simulink model "determinarTiemposYDistanciasEnAceleracion"  (R2017a)
settings: Solver=FixedStepAuto  StartTime=0.0  StopTime=15  FixedStep=0.001  RelTol=1e-3
values from neighbouring files (symbols this model uses):
  vmaxh = 3    [operacionAutomatica.m]
  vmaxt = 4    [operacionAutomatica.m]
undefined symbols (not defined in the file or in its folder): vmaxhfull
settings Model: Creator=yellow submarine  LastModifiedBy=yellow submarine

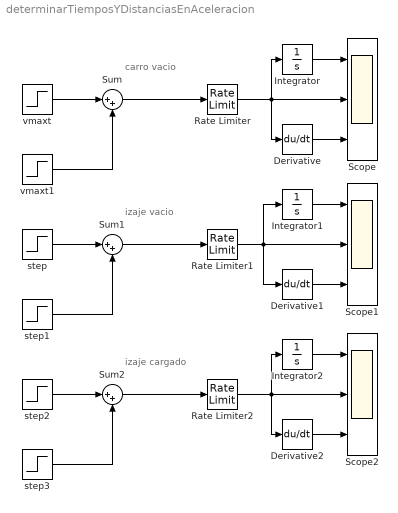
== system determinarTiemposYDistanciasEnAceleracion ==
  note: carro vacio
  note: izaje vacio
  note: izaje cargado
  Derivative : Derivative
  Derivative1 : Derivative
  Derivative2 : Derivative
  Integrator : Integrator
  Integrator1 : Integrator
  Integrator2 : Integrator
  Rate Limiter : RateLimiter
  Rate Limiter1 : RateLimiter
  Rate Limiter2 : RateLimiter
  Scope : Scope  NumInputPorts=3
  Scope1 : Scope  NumInputPorts=3
  Scope2 : Scope  NumInputPorts=3
  Sum : Sum  Inputs=|++
  Sum1 : Sum  Inputs=|++
  Sum2 : Sum  Inputs=|++
  step : Step  Time=.1  After=vmaxh  SampleTime=0
  step1 : Step  Time=3.1  After=-vmaxh  SampleTime=0
  step2 : Step  Time=.1  After=vmaxhfull  SampleTime=0
  step3 : Step  Time=1.6  After=-vmaxhfull  SampleTime=0
  vmaxt : Step  Time=.1  After=vmaxt  SampleTime=0
  vmaxt1 : Step  Time=4.1  After=-vmaxt  SampleTime=0
  wires:
  Sum/1 -> Rate Limiter/1
  vmaxt/1 -> Sum/1
  vmaxt1/1 -> Sum/2
  Rate Limiter/1 -> Integrator/1, Derivative/1, Scope/2
  Derivative/1 -> Scope/3
  step1/1 -> Sum1/2
  step/1 -> Sum1/1
  Sum1/1 -> Rate Limiter1/1
  step2/1 -> Sum2/1
  step3/1 -> Sum2/2
  Sum2/1 -> Rate Limiter2/1
  Integrator/1 -> Scope/1
  Derivative1/1 -> Scope1/3
  Rate Limiter1/1 -> Scope1/2, Derivative1/1, Integrator1/1
  Integrator1/1 -> Scope1/1
  Derivative2/1 -> Scope2/3
  Rate Limiter2/1 -> Integrator2/1, Derivative2/1, Scope2/2
  Integrator2/1 -> Scope2/1
